simulink model "sampleModel7293_pp_1_1"  (R2018a)
settings: Solver=VariableStepAuto  StartTime=0.0  StopTime=10.0  RelTol=1e-3
undefined symbols (not defined in the file): DiscIntNeverNeededParam
libraries: simulink x367
(part 8 of 12)

== system sampleModel7293_pp_1_1/cfblk185/cfblk19 ==
  cfblk1 : Inport
  Action Port : ActionPort  ActionType=else
  cfblk3 : Delay  DelayLengthSource=Input port
      settings: InputPortMap=u0,p1
  cfblk4 : Subsystem  TreatAsAtomicUnit=on
  cfblk5 : DiscreteFir
  cfblk6 : simulink/Discrete/Transfer Fcn Lead or Lag  PoleZ=0.95  ZeroZ=0.75  ICPrevOutput=0.0  ICPrevInput=0.0  DoSatur=off
      settings: SourceProductName=Simulink  SourceProductBaseCode=SL
  cfblk7 : Subsystem  TreatAsAtomicUnit=on
  cfblk8 : Delay
  cyemi_{608..615} (8 alike) : DataTypeConversion  OutDataTypeStr=double
  emi_1381 : Subsystem  TreatAsAtomicUnit=on
  emi_1383 : If  IfExpression=0 <= u1
  emi_1384 : DataTypeConversion  OutDataTypeStr=double
  emi_1759 : Subsystem  TreatAsAtomicUnit=on
  emi_1761 : If  IfExpression=0 <= u1
  emi_1762 : DataTypeConversion  OutDataTypeStr=double
  cfblk2 : Outport
  wires:
  cfblk6/1 -> cfblk2/1, cyemi_611/1
  cfblk1/1 -> cyemi_613/1, cyemi_614/1
  cyemi_608/1 -> cfblk3/1
  cfblk8/1 -> cyemi_608/1, emi_1384/1
  cyemi_609/1 -> cfblk3/2
  cfblk3/1 -> cyemi_610/1
  cyemi_612/1 -> cfblk5/1
  cyemi_613/1 -> cfblk6/1
  cyemi_615/1 -> cfblk8/1
  cfblk5/1 -> cyemi_615/1, emi_1762/1
  cyemi_614/1 -> cfblk7/1(emi_1379)
  cfblk7/1(emi_1380) -> cyemi_609/1
  emi_1383/1 -> cfblk7/Action
  emi_1383/2 -> emi_1381/Action
  emi_1384/1 -> emi_1383/1
  cyemi_610/1 -> cfblk4/1(emi_1756)
  cyemi_611/1 -> cfblk4/2(emi_1757)
  cfblk4/1(emi_1758) -> cyemi_612/1
  emi_1761/1 -> cfblk4/Action
  emi_1761/2 -> emi_1759/Action
  emi_1762/1 -> emi_1761/1

== system sampleModel7293_pp_1_1/cfblk187/cfblk11 ==
  cfblk1 : Inport
  cfblk13 : Inport  Port=2
  cfblk14 : Inport  Port=3
  Action Port : ActionPort  ActionType=then
  cfblk10 : DiscreteFir
  cfblk11 : Delay  ShowEnablePort=on
      settings: InputPortMap=u0,e6
  cfblk12 : Subsystem  TreatAsAtomicUnit=on
  cfblk15 : Subsystem  TreatAsAtomicUnit=on
  cfblk3 : Subsystem  TreatAsAtomicUnit=on
  cfblk4 : Delay
  cfblk5 : DiscreteIntegrator  SampleTime=-1  OutDataTypeStr=double  ICPrevOutput=DiscIntNeverNeededParam  ICPrevScaledInput=DiscIntNeverNeededParam
  cfblk6 : UnitDelay  SampleTime=-1
  cfblk7 : DiscreteTransferFcn
  cfblk8 : simulink/Discrete/Transfer Fcn Lead or Lag  PoleZ=0.95  ZeroZ=0.75  ICPrevOutput=0.0  ICPrevInput=0.0  DoSatur=off
      settings: SourceProductName=Simulink  SourceProductBaseCode=SL
  cfblk9 : Subsystem  TreatAsAtomicUnit=on
  cyemi_{639..650} (12 alike) : DataTypeConversion  OutDataTypeStr=double
  emi_1353 : Subsystem  TreatAsAtomicUnit=on
  emi_{722,1355,1540,2009} (4 alike) : If  IfExpression=Inf <= u1
  emi_{723,1356,1541,2010} (4 alike) : DataTypeConversion  OutDataTypeStr=double
  emi_1538 : Subsystem  TreatAsAtomicUnit=on
  emi_2007 : Subsystem  TreatAsAtomicUnit=on
  emi_720 : Subsystem  TreatAsAtomicUnit=on
  cfblk2 : Outport
  wires:
  cfblk8/1 -> cfblk2/1
  cyemi_639/1 -> cfblk10/1
  cfblk11/1 -> cyemi_639/1, emi_1356/1
  cyemi_640/1 -> cfblk11/1
  cfblk6/1 -> cyemi_640/1
  cyemi_641/1 -> cfblk11/2
  cfblk5/1 -> cyemi_641/1, emi_1541/1
  cfblk7/1 -> cyemi_643/1
  cyemi_645/1 -> cfblk4/1
  cfblk13/1 -> cyemi_645/1
  cyemi_646/1 -> cfblk5/1
  cyemi_647/1 -> cfblk6/1
  cfblk1/1 -> cyemi_647/1
  cyemi_648/1 -> cfblk7/1
  cyemi_649/1 -> cfblk8/1
  cfblk14/1 -> cyemi_649/1
  cfblk4/1 -> cyemi_650/1
  cyemi_643/1 -> cfblk15/1(emi_718)
  cfblk15/1(emi_719) -> cyemi_644/1, emi_2010/1
  emi_722/1 -> cfblk15/Action
  emi_722/2 -> emi_720/Action
  emi_723/1 -> emi_722/1
  cyemi_642/1 -> cfblk12/1(emi_1351)
  cfblk12/1(emi_1352) -> cyemi_646/1
  emi_1355/1 -> cfblk12/Action
  emi_1355/2 -> emi_1353/Action
  emi_1356/1 -> emi_1355/1
  cyemi_650/1 -> cfblk9/1(emi_1536)
  cfblk9/1(emi_1537) -> cyemi_642/1
  emi_1540/1 -> cfblk9/Action
  emi_1540/2 -> emi_1538/Action
  emi_1541/1 -> emi_1540/1
  cyemi_644/1 -> cfblk3/1(emi_2005)
  cfblk3/1(emi_2006) -> emi_723/1, cyemi_648/1
  emi_2009/1 -> cfblk3/Action
  emi_2009/2 -> emi_2007/Action
  emi_2010/1 -> emi_2009/1

== system sampleModel7293_pp_1_1/cfblk187/cfblk12 ==
  cfblk1 : Inport
  cfblk8 : Inport  Port=2
  cfblk9 : Inport  Port=3
  Action Port : ActionPort  ActionType=else
  cfblk3 : Subsystem  TreatAsAtomicUnit=on
  cfblk4 : DiscreteIntegrator  SampleTime=-1  OutDataTypeStr=double  ICPrevOutput=DiscIntNeverNeededParam  ICPrevScaledInput=DiscIntNeverNeededParam
  cfblk5 : Delay
  cfblk6 : DiscreteZeroPole  Poles=[0 0.5]  Gain=1  SampleTime=-1
  cfblk7 : Subsystem  TreatAsAtomicUnit=on
  cyemi_{654..659} (6 alike) : DataTypeConversion  OutDataTypeStr=double
  emi_1190 : Subsystem  TreatAsAtomicUnit=on
  emi_1192 : If  IfExpression=0 <= u1
  emi_1193 : DataTypeConversion  OutDataTypeStr=double
  emi_324 : Subsystem  TreatAsAtomicUnit=on
  emi_326 : If  IfExpression=0 <= u1
  emi_327 : DataTypeConversion  OutDataTypeStr=double
  cfblk2 : Outport
  cfblk10 : Outport  Port=2
  wires:
  cfblk5/1 -> cfblk2/1
  cfblk8/1 -> cfblk10/1
  cfblk1/1 -> cyemi_654/1
  cfblk6/1 -> cyemi_655/1, emi_327/1
  cyemi_656/1 -> cfblk4/1
  cyemi_657/1 -> cfblk5/1
  cyemi_658/1 -> cfblk6/1
  cfblk4/1 -> cyemi_658/1, emi_1193/1
  cfblk9/1 -> cyemi_659/1
  cyemi_659/1 -> cfblk7/1(emi_322)
  cfblk7/1(emi_323) -> cyemi_656/1
  emi_326/1 -> cfblk7/Action
  emi_326/2 -> emi_324/Action
  emi_327/1 -> emi_326/1
  cyemi_654/1 -> cfblk3/1(emi_1187)
  cyemi_655/1 -> cfblk3/2(emi_1188)
  cfblk3/1(emi_1189) -> cyemi_657/1
  emi_1192/1 -> cfblk3/Action
  emi_1192/2 -> emi_1190/Action
  emi_1193/1 -> emi_1192/1

== system sampleModel7293_pp_1_1/cfblk187/cfblk14 ==
  emi_774 : Inport
  Action Port : ActionPort  ActionType=then
  cfblk14 : Delay
  emi_775 : Outport
  wires:
  emi_774/1 -> cfblk14/1
  cfblk14/1 -> emi_775/1

== system sampleModel7293_pp_1_1/cfblk187/cfblk3 ==
  emi_336 : Inport
  emi_337 : Inport  Port=2
  Action Port : ActionPort  ActionType=then
  cfblk3 : simulink/Continuous/PID Controller (2DOF)  Controller=PID  TimeDomain=Discrete-time  SampleTime=-1  IntegratorMethod=Forward Euler  FilterMethod=Forward Euler  Form=Parallel  UseFilter=on  ControllerParametersSource=internal  P=1  I=1  D=0  N=100  b=1  c=1  InitialConditionSource=internal  InitialConditionForIntegrator=0  InitialConditionForFilter=0  ExternalReset=none  LimitOutput=off  UpperSaturationLimit=inf  LowerSaturationLimit=-inf  LinearizeAsGain=off  AntiWindupMode=none  Kb=1  TrackingMode=off  Kt=1  PParamMin=[]  PParamMax=[]  IParamMin=[]  IParamMax=[]  DParamMin=[]  DParamMax=[]  NParamMin=[]  NParamMax=[]  bParamMin=[]  bParamMax=[]  cParamMin=[]  cParamMax=[]  KbParamMin=[]  KbParamMax=[]  KtParamMin=[]  KtParamMax=[]  POutMin=[]  POutMax=[]  IOutMin=[]  IOutMax=[]  DOutMin=[]  DOutMax=[]  NOutMin=[]  NOutMax=[]  bOutMin=[]  bOutMax=[]  cOutMin=[]  cOutMax=[]  KbOutMin=[]  KbOutMax=[]  KtOutMin=[]  KtOutMax=[]  IntegratorOutMin=[]  IntegratorOutMax=[]  FilterOutMin=[]  FilterOutMax=[]  SumOutMin=[]  SumOutMax=[]  Sum1OutMin=[]  Sum1OutMax=[]  Sum2OutMin=[]  Sum2OutMax=[]  Sum3OutMin=[]  Sum3OutMax=[]  SumI1OutMin=[]  SumI1OutMax=[]  SumI2OutMin=[]  SumI2OutMax=[]  SumI3OutMin=[]  SumI3OutMax=[]  SumDOutMin=[]  SumDOutMax=[]  SaturationOutMin=[]  SaturationOutMax=[]  IntegratorContinuousStateAttributes=''  IntegratorStateMustResolveToSignalObject=off  IntegratorRTWStateStorageClass=Auto  FilterContinuousStateAttributes=''  FilterStateMustResolveToSignalObject=off  FilterRTWStateStorageClass=Auto  DifferentiatorICPrevScaledInput=0  DifferentiatorOutMin=[]  DifferentiatorOutMax=[]  FilterDiffOutCoefMin=[]  FilterDiffOutCoefMax=[]  SumDenOutMin=[]  SumDenOutMax=[]  SumNumOutMin=[]  SumNumOutMax=[]  ReciprocalOutMin=[]  ReciprocalOutMax=[]  DivideOutMin=[]  DivideOutMax=[]  TunerSelectOption=Transfer Function Based (PID Tuner App)
  emi_338 : Outport
  wires:
  emi_336/1 -> cfblk3/1
  emi_337/1 -> cfblk3/2
  cfblk3/1 -> emi_338/1

== system sampleModel7293_pp_1_1/cfblk187/emi_339 ==
  Action Port : ActionPort  ActionType=else
  emi_340 : Assertion

== system sampleModel7293_pp_1_1/cfblk187/emi_776 ==
  Action Port : ActionPort  ActionType=else
  emi_777 : Assertion

== system sampleModel7293_pp_1_1/cfblk188/cfblk3 ==
  emi_646 : Inport
  Action Port : ActionPort  ActionType=then
  cfblk3 : DiscreteTransferFcn
  emi_647 : Outport
  wires:
  emi_646/1 -> cfblk3/1
  cfblk3/1 -> emi_647/1

== system sampleModel7293_pp_1_1/cfblk188/cfblk4 ==
  emi_1471 : Inport
  Action Port : ActionPort  ActionType=then
  cfblk4 : DiscreteFir
  emi_1472 : Outport
  wires:
  emi_1471/1 -> cfblk4/1
  cfblk4/1 -> emi_1472/1

== system sampleModel7293_pp_1_1/cfblk188/cfblk5 ==
  emi_450 : Inport
  Action Port : ActionPort  ActionType=then
  cfblk5 : DiscreteZeroPole  Poles=[0 0.5]  Gain=1  SampleTime=-1
  emi_451 : Outport
  wires:
  emi_450/1 -> cfblk5/1
  cfblk5/1 -> emi_451/1

== system sampleModel7293_pp_1_1/cfblk188/cfblk6 ==
  emi_178 : Inport
  Action Port : ActionPort  ActionType=then
  cfblk6 : simulink/Discrete/Transfer Fcn First Order  PoleZ=0.95  ICPrevOutput=0.0  DoSatur=off
      settings: SourceProductName=Simulink
  emi_179 : Outport
  wires:
  emi_178/1 -> cfblk6/1
  cfblk6/1 -> emi_179/1

== system sampleModel7293_pp_1_1/cfblk188/emi_1473 ==
  Action Port : ActionPort  ActionType=else
  emi_1474 : Assertion

== system sampleModel7293_pp_1_1/cfblk188/emi_180 ==
  Action Port : ActionPort  ActionType=else
  emi_181 : Assertion

== system sampleModel7293_pp_1_1/cfblk188/emi_452 ==
  Action Port : ActionPort  ActionType=else
  emi_453 : Assertion

== system sampleModel7293_pp_1_1/cfblk188/emi_648 ==
  Action Port : ActionPort  ActionType=else
  emi_649 : Assertion

== system sampleModel7293_pp_1_1/cfblk189/cfblk16 ==
  cfblk1 : Inport
  cfblk11 : Inport  Port=2
  cfblk12 : Inport  Port=3
  cfblk13 : Inport  Port=4
  Action Port : ActionPort  ActionType=then
  cfblk10 : simulink/Continuous/PID Controller (2DOF)  Controller=PID  TimeDomain=Discrete-time  SampleTime=-1  IntegratorMethod=Forward Euler  FilterMethod=Forward Euler  Form=Parallel  UseFilter=on  ControllerParametersSource=internal  P=1  I=1  D=0  N=100  b=1  c=1  InitialConditionSource=internal  InitialConditionForIntegrator=0  InitialConditionForFilter=0  ExternalReset=none  LimitOutput=off  UpperSaturationLimit=inf  LowerSaturationLimit=-inf  LinearizeAsGain=off  AntiWindupMode=none  Kb=1  TrackingMode=off  Kt=1  PParamMin=[]  PParamMax=[]  IParamMin=[]  IParamMax=[]  DParamMin=[]  DParamMax=[]  NParamMin=[]  NParamMax=[]  bParamMin=[]  bParamMax=[]  cParamMin=[]  cParamMax=[]  KbParamMin=[]  KbParamMax=[]  KtParamMin=[]  KtParamMax=[]  POutMin=[]  POutMax=[]  IOutMin=[]  IOutMax=[]  DOutMin=[]  DOutMax=[]  NOutMin=[]  NOutMax=[]  bOutMin=[]  bOutMax=[]  cOutMin=[]  cOutMax=[]  KbOutMin=[]  KbOutMax=[]  KtOutMin=[]  KtOutMax=[]  IntegratorOutMin=[]  IntegratorOutMax=[]  FilterOutMin=[]  FilterOutMax=[]  SumOutMin=[]  SumOutMax=[]  Sum1OutMin=[]  Sum1OutMax=[]  Sum2OutMin=[]  Sum2OutMax=[]  Sum3OutMin=[]  Sum3OutMax=[]  SumI1OutMin=[]  SumI1OutMax=[]  SumI2OutMin=[]  SumI2OutMax=[]  SumI3OutMin=[]  SumI3OutMax=[]  SumDOutMin=[]  SumDOutMax=[]  SaturationOutMin=[]  SaturationOutMax=[]  IntegratorContinuousStateAttributes=''  IntegratorStateMustResolveToSignalObject=off  IntegratorRTWStateStorageClass=Auto  FilterContinuousStateAttributes=''  FilterStateMustResolveToSignalObject=off  FilterRTWStateStorageClass=Auto  DifferentiatorICPrevScaledInput=0  DifferentiatorOutMin=[]  DifferentiatorOutMax=[]  FilterDiffOutCoefMin=[]  FilterDiffOutCoefMax=[]  SumDenOutMin=[]  SumDenOutMax=[]  SumNumOutMin=[]  SumNumOutMax=[]  ReciprocalOutMin=[]  ReciprocalOutMax=[]  DivideOutMin=[]  DivideOutMax=[]  TunerSelectOption=Transfer Function Based (PID Tuner App)
  cfblk3 : DiscreteFilter
  cfblk4 : simulink/Discrete/Transfer Fcn Real Zero  ZeroZ=0.75  ICPrevInput=0.0  DoSatur=off
      settings: SourceProductName=Simulink  SourceProductBaseCode=SL
  cfblk5 : simulink/Discrete/Tapped Delay  vinit=0.0  samptime=-1  NumDelays=1  DelayOrder=Oldest  includeCurrent=off
  cfblk6 : simulink/Discrete/Difference  ICPrevInput=0.0  OutMin=[]  OutMax=[]  OutDataTypeStr=double  OutputDataTypeScalingMode=double  OutDataType=fixdt(1, 16)  OutScaling=2^-10  DoSatur=off
  cfblk7 : simulink/Discrete/Transfer Fcn Lead or Lag  PoleZ=0.95  ZeroZ=0.75  ICPrevOutput=0.0  ICPrevInput=0.0  DoSatur=off
      settings: SourceProductName=Simulink  SourceProductBaseCode=SL
  cfblk8 : Subsystem  TreatAsAtomicUnit=on
  cfblk9 : DiscreteZeroPole  Poles=[0 0.5]  Gain=1  SampleTime=-1
  cyemi_{690..698} (9 alike) : DataTypeConversion  OutDataTypeStr=double
  emi_905 : Subsystem  TreatAsAtomicUnit=on
  emi_907 : If  IfExpression=0 <= u1
  emi_908 : DataTypeConversion  OutDataTypeStr=double
  cfblk2 : Outport
  wires:
  cfblk9/1 -> cfblk2/1
  cyemi_690/1 -> cfblk10/1
  cfblk6/1 -> cyemi_690/1
  cyemi_691/1 -> cfblk10/2
  cfblk7/1 -> cyemi_691/1
  cyemi_692/1 -> cfblk3/1
  cfblk12/1 -> cyemi_692/1
  cyemi_693/1 -> cfblk4/1
  cfblk11/1 -> cyemi_693/1
  cyemi_694/1 -> cfblk5/1
  cfblk4/1 -> cyemi_694/1
  cyemi_695/1 -> cfblk6/1
  cyemi_696/1 -> cfblk7/1
  cfblk13/1 -> cyemi_696/1
  cfblk3/1 -> cyemi_697/1, emi_908/1
  cyemi_698/1 -> cfblk9/1
  cfblk1/1 -> cyemi_698/1
  cyemi_697/1 -> cfblk8/1(emi_903)
  cfblk8/1(emi_904) -> cyemi_695/1
  emi_907/1 -> cfblk8/Action
  emi_907/2 -> emi_905/Action
  emi_908/1 -> emi_907/1

== system sampleModel7293_pp_1_1/cfblk189/cfblk17 ==
  cfblk1 : Inport
  cfblk15 : Inport  Port=2
  Action Port : ActionPort  ActionType=else
  cfblk10 : simulink/Continuous/PID Controller  Controller=PID  TimeDomain=Discrete-time  SampleTime=-1  IntegratorMethod=Forward Euler  FilterMethod=Forward Euler  Form=Parallel  UseFilter=on  ControllerParametersSource=internal  P=1  I=1  D=0  N=100  InitialConditionSource=internal  InitialConditionForIntegrator=0  InitialConditionForFilter=0  ExternalReset=none  LimitOutput=off  UpperSaturationLimit=inf  LowerSaturationLimit=-inf  LinearizeAsGain=off  AntiWindupMode=none  Kb=1  TrackingMode=off  Kt=1  PParamMin=[]  PParamMax=[]  IParamMin=[]  IParamMax=[]  DParamMin=[]  DParamMax=[]  NParamMin=[]  NParamMax=[]  KbParamMin=[]  KbParamMax=[]  KtParamMin=[]  KtParamMax=[]  POutMin=[]  POutMax=[]  IOutMin=[]  IOutMax=[]  DOutMin=[]  DOutMax=[]  NOutMin=[]  NOutMax=[]  KbOutMin=[]  KbOutMax=[]  KtOutMin=[]  KtOutMax=[]  IntegratorOutMin=[]  IntegratorOutMax=[]  FilterOutMin=[]  FilterOutMax=[]  SumOutMin=[]  SumOutMax=[]  SumI1OutMin=[]  SumI1OutMax=[]  SumI2OutMin=[]  SumI2OutMax=[]  SumI3OutMin=[]  SumI3OutMax=[]  SumDOutMin=[]  SumDOutMax=[]  SaturationOutMin=[]  SaturationOutMax=[]  IntegratorContinuousStateAttributes=''  IntegratorStateMustResolveToSignalObject=off  IntegratorRTWStateStorageClass=Auto  FilterContinuousStateAttributes=''  FilterStateMustResolveToSignalObject=off  FilterRTWStateStorageClass=Auto  DifferentiatorICPrevScaledInput=0  DifferentiatorOutMin=[]  DifferentiatorOutMax=[]  FilterDiffOutCoefMin=[]  FilterDiffOutCoefMax=[]  SumDenOutMin=[]  SumDenOutMax=[]  SumNumOutMin=[]  SumNumOutMax=[]  ReciprocalOutMin=[]  ReciprocalOutMax=[]  DivideOutMin=[]  DivideOutMax=[]  TunerSelectOption=Transfer Function Based (PID Tuner App)
  cfblk11 : simulink/Discrete/Tapped Delay  vinit=0.0  samptime=-1  NumDelays=1  DelayOrder=Oldest  includeCurrent=off
  cfblk12 : DiscreteFilter
  cfblk13 : Subsystem  TreatAsAtomicUnit=on
  cfblk14 : DiscreteStateSpace  SampleTime=-1
  cfblk16 : Delay
  cfblk17 : DataTypeConversion  OutDataTypeStr=uint32
  cfblk3 : DiscreteTransferFcn
  cfblk4 : Subsystem  TreatAsAtomicUnit=on
  cfblk5 : Delay  ShowEnablePort=on
      settings: InputPortMap=u0,e6
  cfblk6 : simulink/Discrete/Transfer Fcn Lead or Lag  PoleZ=0.95  ZeroZ=0.75  ICPrevOutput=0.0  ICPrevInput=0.0  DoSatur=off
      settings: SourceProductName=Simulink  SourceProductBaseCode=SL
  cfblk7 : simulink/Continuous/PID Controller  Controller=PID  TimeDomain=Discrete-time  SampleTime=-1  IntegratorMethod=Forward Euler  FilterMethod=Forward Euler  Form=Parallel  UseFilter=on  ControllerParametersSource=internal  P=1  I=1  D=0  N=100  InitialConditionSource=internal  InitialConditionForIntegrator=0  InitialConditionForFilter=0  ExternalReset=none  LimitOutput=off  UpperSaturationLimit=inf  LowerSaturationLimit=-inf  LinearizeAsGain=off  AntiWindupMode=none  Kb=1  TrackingMode=off  Kt=1  PParamMin=[]  PParamMax=[]  IParamMin=[]  IParamMax=[]  DParamMin=[]  DParamMax=[]  NParamMin=[]  NParamMax=[]  KbParamMin=[]  KbParamMax=[]  KtParamMin=[]  KtParamMax=[]  POutMin=[]  POutMax=[]  IOutMin=[]  IOutMax=[]  DOutMin=[]  DOutMax=[]  NOutMin=[]  NOutMax=[]  KbOutMin=[]  KbOutMax=[]  KtOutMin=[]  KtOutMax=[]  IntegratorOutMin=[]  IntegratorOutMax=[]  FilterOutMin=[]  FilterOutMax=[]  SumOutMin=[]  SumOutMax=[]  SumI1OutMin=[]  SumI1OutMax=[]  SumI2OutMin=[]  SumI2OutMax=[]  SumI3OutMin=[]  SumI3OutMax=[]  SumDOutMin=[]  SumDOutMax=[]  SaturationOutMin=[]  SaturationOutMax=[]  IntegratorContinuousStateAttributes=''  IntegratorStateMustResolveToSignalObject=off  IntegratorRTWStateStorageClass=Auto  FilterContinuousStateAttributes=''  FilterStateMustResolveToSignalObject=off  FilterRTWStateStorageClass=Auto  DifferentiatorICPrevScaledInput=0  DifferentiatorOutMin=[]  DifferentiatorOutMax=[]  FilterDiffOutCoefMin=[]  FilterDiffOutCoefMax=[]  SumDenOutMin=[]  SumDenOutMax=[]  SumNumOutMin=[]  SumNumOutMax=[]  ReciprocalOutMin=[]  ReciprocalOutMax=[]  DivideOutMin=[]  DivideOutMax=[]  TunerSelectOption=Transfer Function Based (PID Tuner App)
  cfblk8 : simulink/Continuous/PID Controller  Controller=PID  TimeDomain=Discrete-time  SampleTime=-1  IntegratorMethod=Forward Euler  FilterMethod=Forward Euler  Form=Parallel  UseFilter=on  ControllerParametersSource=internal  P=1  I=1  D=0  N=100  InitialConditionSource=internal  InitialConditionForIntegrator=0  InitialConditionForFilter=0  ExternalReset=none  LimitOutput=off  UpperSaturationLimit=inf  LowerSaturationLimit=-inf  LinearizeAsGain=off  AntiWindupMode=none  Kb=1  TrackingMode=off  Kt=1  PParamMin=[]  PParamMax=[]  IParamMin=[]  IParamMax=[]  DParamMin=[]  DParamMax=[]  NParamMin=[]  NParamMax=[]  KbParamMin=[]  KbParamMax=[]  KtParamMin=[]  KtParamMax=[]  POutMin=[]  POutMax=[]  IOutMin=[]  IOutMax=[]  DOutMin=[]  DOutMax=[]  NOutMin=[]  NOutMax=[]  KbOutMin=[]  KbOutMax=[]  KtOutMin=[]  KtOutMax=[]  IntegratorOutMin=[]  IntegratorOutMax=[]  FilterOutMin=[]  FilterOutMax=[]  SumOutMin=[]  SumOutMax=[]  SumI1OutMin=[]  SumI1OutMax=[]  SumI2OutMin=[]  SumI2OutMax=[]  SumI3OutMin=[]  SumI3OutMax=[]  SumDOutMin=[]  SumDOutMax=[]  SaturationOutMin=[]  SaturationOutMax=[]  IntegratorContinuousStateAttributes=''  IntegratorStateMustResolveToSignalObject=off  IntegratorRTWStateStorageClass=Auto  FilterContinuousStateAttributes=''  FilterStateMustResolveToSignalObject=off  FilterRTWStateStorageClass=Auto  DifferentiatorICPrevScaledInput=0  DifferentiatorOutMin=[]  DifferentiatorOutMax=[]  FilterDiffOutCoefMin=[]  FilterDiffOutCoefMax=[]  SumDenOutMin=[]  SumDenOutMax=[]  SumNumOutMin=[]  SumNumOutMax=[]  ReciprocalOutMin=[]  ReciprocalOutMax=[]  DivideOutMin=[]  DivideOutMax=[]  TunerSelectOption=Transfer Function Based (PID Tuner App)
  cfblk9 : Subsystem  TreatAsAtomicUnit=on
  cyemi_{701..715} (15 alike) : DataTypeConversion  OutDataTypeStr=double
  emi_361 : Subsystem  TreatAsAtomicUnit=on
  emi_363 : If  IfExpression=0 <= u1
  emi_364 : DataTypeConversion  OutDataTypeStr=double
  emi_368 : Subsystem  TreatAsAtomicUnit=on
  emi_370 : If  IfExpression=0 <= u1
  emi_371 : DataTypeConversion  OutDataTypeStr=double
  emi_812 : Subsystem  TreatAsAtomicUnit=on
  emi_814 : If  IfExpression=0 <= u1
  emi_815 : DataTypeConversion  OutDataTypeStr=double
  cfblk2 : Outport
  wires:
  cfblk17/1 -> cfblk2/1
  cyemi_701/1 -> cfblk10/1
  cfblk11/1 -> cyemi_701/1, emi_815/1
  cyemi_702/1 -> cfblk11/1
  cfblk12/1 -> cyemi_702/1
  cyemi_703/1 -> cfblk12/1
  cfblk7/1 -> cyemi_703/1
  cfblk10/1 -> cyemi_704/1
  cyemi_705/1 -> cfblk14/1
  cfblk15/1 -> cyemi_705/1
  cyemi_706/1 -> cfblk16/1
  cyemi_707/1 -> cfblk17/1
  cyemi_708/1 -> cfblk3/1
  cfblk8/1 -> cyemi_708/1
  cfblk14/1 -> cyemi_709/1
  cyemi_710/1 -> cfblk5/1
  cyemi_711/1 -> cfblk5/2
  cfblk16/1 -> cyemi_711/1
  cyemi_712/1 -> cfblk6/1
  cfblk5/1 -> cyemi_712/1
  cyemi_713/1 -> cfblk7/1
  cfblk6/1 -> cyemi_713/1
  cyemi_714/1 -> cfblk8/1
  cfblk1/1 -> cyemi_714/1
  cfblk3/1 -> cyemi_715/1, emi_364/1, emi_371/1
  cyemi_704/1 -> cfblk13/1(emi_359)
  cfblk13/1(emi_360) -> cyemi_706/1
  emi_363/1 -> cfblk13/Action
  emi_363/2 -> emi_361/Action
  emi_364/1 -> emi_363/1
  cyemi_715/1 -> cfblk9/1(emi_366)
  cfblk9/1(emi_367) -> cyemi_710/1
  emi_370/1 -> cfblk9/Action
  emi_370/2 -> emi_368/Action
  emi_371/1 -> emi_370/1
  cyemi_709/1 -> cfblk4/1(emi_810)
  cfblk4/1(emi_811) -> cyemi_707/1
  emi_814/1 -> cfblk4/Action
  emi_814/2 -> emi_812/Action
  emi_815/1 -> emi_814/1

== system sampleModel7293_pp_1_1/cfblk189/cfblk4 ==
  emi_1237 : Inport
  emi_1238 : Inport  Port=2
  Action Port : ActionPort  ActionType=then
  cfblk4 : simulink/Continuous/PID Controller (2DOF)  Controller=PID  TimeDomain=Discrete-time  SampleTime=-1  IntegratorMethod=Forward Euler  FilterMethod=Forward Euler  Form=Parallel  UseFilter=on  ControllerParametersSource=internal  P=1  I=1  D=0  N=100  b=1  c=1  InitialConditionSource=internal  InitialConditionForIntegrator=0  InitialConditionForFilter=0  ExternalReset=none  LimitOutput=off  UpperSaturationLimit=inf  LowerSaturationLimit=-inf  LinearizeAsGain=off  AntiWindupMode=none  Kb=1  TrackingMode=off  Kt=1  PParamMin=[]  PParamMax=[]  IParamMin=[]  IParamMax=[]  DParamMin=[]  DParamMax=[]  NParamMin=[]  NParamMax=[]  bParamMin=[]  bParamMax=[]  cParamMin=[]  cParamMax=[]  KbParamMin=[]  KbParamMax=[]  KtParamMin=[]  KtParamMax=[]  POutMin=[]  POutMax=[]  IOutMin=[]  IOutMax=[]  DOutMin=[]  DOutMax=[]  NOutMin=[]  NOutMax=[]  bOutMin=[]  bOutMax=[]  cOutMin=[]  cOutMax=[]  KbOutMin=[]  KbOutMax=[]  KtOutMin=[]  KtOutMax=[]  IntegratorOutMin=[]  IntegratorOutMax=[]  FilterOutMin=[]  FilterOutMax=[]  SumOutMin=[]  SumOutMax=[]  Sum1OutMin=[]  Sum1OutMax=[]  Sum2OutMin=[]  Sum2OutMax=[]  Sum3OutMin=[]  Sum3OutMax=[]  SumI1OutMin=[]  SumI1OutMax=[]  SumI2OutMin=[]  SumI2OutMax=[]  SumI3OutMin=[]  SumI3OutMax=[]  SumDOutMin=[]  SumDOutMax=[]  SaturationOutMin=[]  SaturationOutMax=[]  IntegratorContinuousStateAttributes=''  IntegratorStateMustResolveToSignalObject=off  IntegratorRTWStateStorageClass=Auto  FilterContinuousStateAttributes=''  FilterStateMustResolveToSignalObject=off  FilterRTWStateStorageClass=Auto  DifferentiatorICPrevScaledInput=0  DifferentiatorOutMin=[]  DifferentiatorOutMax=[]  FilterDiffOutCoefMin=[]  FilterDiffOutCoefMax=[]  SumDenOutMin=[]  SumDenOutMax=[]  SumNumOutMin=[]  SumNumOutMax=[]  ReciprocalOutMin=[]  ReciprocalOutMax=[]  DivideOutMin=[]  DivideOutMax=[]  TunerSelectOption=Transfer Function Based (PID Tuner App)
  emi_1239 : Outport
  wires:
  emi_1237/1 -> cfblk4/1
  emi_1238/1 -> cfblk4/2
  cfblk4/1 -> emi_1239/1

== system sampleModel7293_pp_1_1/cfblk189/cfblk5 ==
  emi_1508 : Inport
  Action Port : ActionPort  ActionType=then
  cfblk5 : simulink/Discrete/Transfer Fcn Lead or Lag  PoleZ=0.95  ZeroZ=0.75  ICPrevOutput=0.0  ICPrevInput=0.0  DoSatur=off
      settings: SourceProductName=Simulink  SourceProductBaseCode=SL
  emi_1509 : Outport
  wires:
  emi_1508/1 -> cfblk5/1
  cfblk5/1 -> emi_1509/1

== system sampleModel7293_pp_1_1/cfblk189/emi_1240 ==
  Action Port : ActionPort  ActionType=else
  emi_1241 : Assertion

== system sampleModel7293_pp_1_1/cfblk189/emi_1510 ==
  Action Port : ActionPort  ActionType=else
  emi_1511 : Assertion

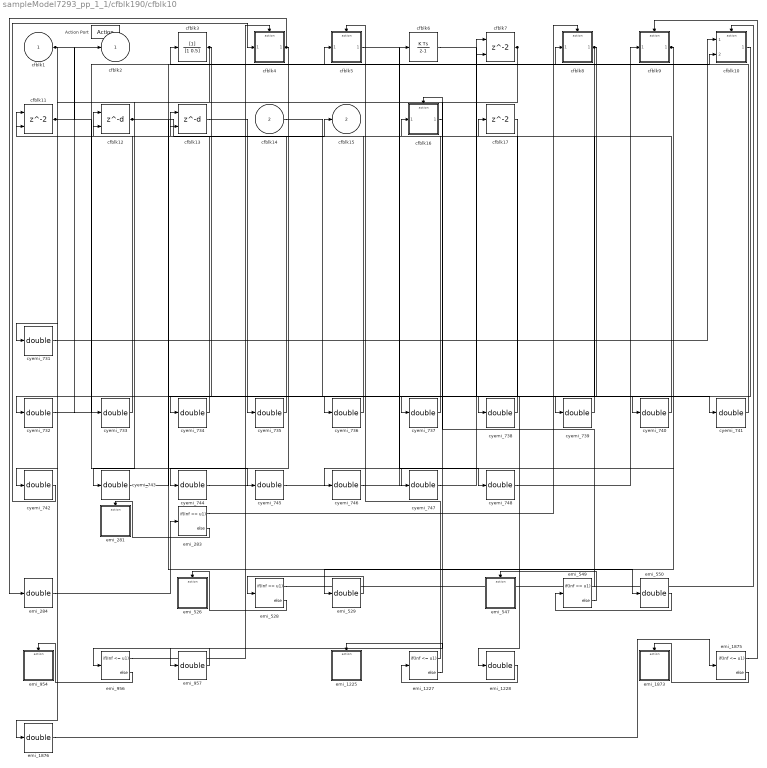
== system sampleModel7293_pp_1_1/cfblk190/cfblk10 ==
  cfblk1 : Inport
  cfblk14 : Inport  Port=2
  Action Port : ActionPort  ActionType=else
  cfblk10 : Subsystem  TreatAsAtomicUnit=on
  cfblk11 : Delay  ShowEnablePort=on
      settings: InputPortMap=u0,e6
  cfblk12 : Delay  DelayLengthSource=Input port
      settings: InputPortMap=u0,p1
  cfblk13 : Delay  DelayLengthSource=Input port
      settings: InputPortMap=u0,p1
  cfblk16 : Subsystem  TreatAsAtomicUnit=on
  cfblk17 : Delay
  cfblk3 : DiscreteFilter
  cfblk4 : Subsystem  TreatAsAtomicUnit=on
  cfblk5 : Subsystem  TreatAsAtomicUnit=on
  cfblk6 : DiscreteIntegrator  SampleTime=-1  OutDataTypeStr=double  ICPrevOutput=DiscIntNeverNeededParam  ICPrevScaledInput=DiscIntNeverNeededParam
  cfblk7 : Delay  ShowEnablePort=on
      settings: InputPortMap=u0,e6
  cfblk8 : Subsystem  TreatAsAtomicUnit=on
  cfblk9 : Subsystem  TreatAsAtomicUnit=on
  cyemi_{731..748} (18 alike) : DataTypeConversion  OutDataTypeStr=double
  emi_1225 : Subsystem  TreatAsAtomicUnit=on
  emi_{283,528,549,956,1227,1875} (6 alike) : If  IfExpression=Inf <= u1
  emi_{284,529,550,957,1228,1876} (6 alike) : DataTypeConversion  OutDataTypeStr=double
  emi_1873 : Subsystem  TreatAsAtomicUnit=on
  emi_281 : Subsystem  TreatAsAtomicUnit=on
  emi_526 : Subsystem  TreatAsAtomicUnit=on
  emi_547 : Subsystem  TreatAsAtomicUnit=on
  emi_954 : Subsystem  TreatAsAtomicUnit=on
  cfblk2 : Outport
  cfblk15 : Outport  Port=2
  wires:
  cfblk11/1 -> cfblk2/1, cyemi_745/1
  cfblk1/1 -> cyemi_731/1, cyemi_733/1
  cfblk3/1 -> cyemi_732/1, cyemi_734/1, emi_1876/1
  cfblk12/1 -> cfblk15/1, cyemi_739/1, emi_550/1
  cyemi_733/1 -> cfblk11/1
  cyemi_734/1 -> cfblk11/2
  cyemi_735/1 -> cfblk12/1
  cfblk13/1 -> cyemi_735/1
  cyemi_736/1 -> cfblk12/2
  cyemi_737/1 -> cfblk13/1
  cyemi_738/1 -> cfblk13/2
  cyemi_740/1 -> cfblk17/1
  cfblk6/1 -> cyemi_740/1
  cyemi_741/1 -> cfblk3/1
  cfblk14/1 -> cyemi_741/1
  cfblk17/1 -> cyemi_742/1
  cfblk7/1 -> cyemi_743/1, emi_957/1
  cyemi_744/1 -> cfblk6/1
  cyemi_745/1 -> cfblk7/1
  cyemi_746/1 -> cfblk7/2
  cyemi_747/1 -> cfblk8/1(emi_279)
  cfblk8/1(emi_280) -> cyemi_737/1, cyemi_736/1, emi_1228/1
  emi_283/1 -> cfblk8/Action
  emi_283/2 -> emi_281/Action
  emi_284/1 -> emi_283/1
  cyemi_731/1 -> cfblk10/1(emi_523)
  cyemi_732/1 -> cfblk10/2(emi_524)
  cfblk10/1(emi_525) -> cyemi_738/1
  emi_528/1 -> cfblk10/Action
  emi_528/2 -> emi_526/Action
  emi_529/1 -> emi_528/1
  cyemi_739/1 -> cfblk16/1(emi_545)
  cfblk16/1(emi_546) -> cyemi_746/1
  emi_549/1 -> cfblk16/Action
  emi_549/2 -> emi_547/Action
  emi_550/1 -> emi_549/1
  cyemi_742/1 -> cfblk4/1(emi_952)
  cfblk4/1(emi_953) -> emi_284/1, cyemi_744/1
  emi_956/1 -> cfblk4/Action
  emi_956/2 -> emi_954/Action
  emi_957/1 -> emi_956/1
  cyemi_743/1 -> cfblk5/1(emi_1223)
  cfblk5/1(emi_1224) -> cyemi_748/1
  emi_1227/1 -> cfblk5/Action
  emi_1227/2 -> emi_1225/Action
  emi_1228/1 -> emi_1227/1
  cyemi_748/1 -> cfblk9/1(emi_1871)
  cfblk9/1(emi_1872) -> emi_529/1, cyemi_747/1
  emi_1875/1 -> cfblk9/Action
  emi_1875/2 -> emi_1873/Action
  emi_1876/1 -> emi_1875/1

== system sampleModel7293_pp_1_1/cfblk190/cfblk12 ==
  emi_2140 : Inport
  Action Port : ActionPort  ActionType=then
  cfblk12 : Delay
  emi_2141 : Outport
  wires:
  emi_2140/1 -> cfblk12/1
  cfblk12/1 -> emi_2141/1

== system sampleModel7293_pp_1_1/cfblk190/cfblk13 ==
  emi_1800 : Inport
  Action Port : ActionPort  ActionType=then
  cfblk13 : Delay
  emi_1801 : Outport
  wires:
  emi_1800/1 -> cfblk13/1
  cfblk13/1 -> emi_1801/1

== system sampleModel7293_pp_1_1/cfblk190/cfblk3 ==
  emi_2026 : Inport
  Action Port : ActionPort  ActionType=then
  cfblk3 : simulink/Discrete/Transfer Fcn Lead or Lag  PoleZ=0.95  ZeroZ=0.75  ICPrevOutput=0.0  ICPrevInput=0.0  DoSatur=off
      settings: SourceProductName=Simulink  SourceProductBaseCode=SL
  emi_2027 : Outport
  wires:
  emi_2026/1 -> cfblk3/1
  cfblk3/1 -> emi_2027/1

== system sampleModel7293_pp_1_1/cfblk190/cfblk5 ==
  emi_917 : Inport
  Action Port : ActionPort  ActionType=then
  cfblk5 : simulink/Discrete/Transfer Fcn Real Zero  ZeroZ=0.75  ICPrevInput=0.0  DoSatur=off
      settings: SourceProductName=Simulink  SourceProductBaseCode=SL
  emi_918 : Outport
  wires:
  emi_917/1 -> cfblk5/1
  cfblk5/1 -> emi_918/1

== system sampleModel7293_pp_1_1/cfblk190/cfblk9 ==
  cfblk1 : Inport
  Action Port : ActionPort  ActionType=then
  cfblk10 : Subsystem  TreatAsAtomicUnit=on
  cfblk11 : DiscreteZeroPole  Poles=[0 0.5]  Gain=1  SampleTime=-1
  cfblk12 : DiscreteTransferFcn
  cfblk13 : simulink/Continuous/PID Controller (2DOF)  Controller=PID  TimeDomain=Discrete-time  SampleTime=-1  IntegratorMethod=Forward Euler  FilterMethod=Forward Euler  Form=Parallel  UseFilter=on  ControllerParametersSource=internal  P=1  I=1  D=0  N=100  b=1  c=1  InitialConditionSource=internal  InitialConditionForIntegrator=0  InitialConditionForFilter=0  ExternalReset=none  LimitOutput=off  UpperSaturationLimit=inf  LowerSaturationLimit=-inf  LinearizeAsGain=off  AntiWindupMode=none  Kb=1  TrackingMode=off  Kt=1  PParamMin=[]  PParamMax=[]  IParamMin=[]  IParamMax=[]  DParamMin=[]  DParamMax=[]  NParamMin=[]  NParamMax=[]  bParamMin=[]  bParamMax=[]  cParamMin=[]  cParamMax=[]  KbParamMin=[]  KbParamMax=[]  KtParamMin=[]  KtParamMax=[]  POutMin=[]  POutMax=[]  IOutMin=[]  IOutMax=[]  DOutMin=[]  DOutMax=[]  NOutMin=[]  NOutMax=[]  bOutMin=[]  bOutMax=[]  cOutMin=[]  cOutMax=[]  KbOutMin=[]  KbOutMax=[]  KtOutMin=[]  KtOutMax=[]  IntegratorOutMin=[]  IntegratorOutMax=[]  FilterOutMin=[]  FilterOutMax=[]  SumOutMin=[]  SumOutMax=[]  Sum1OutMin=[]  Sum1OutMax=[]  Sum2OutMin=[]  Sum2OutMax=[]  Sum3OutMin=[]  Sum3OutMax=[]  SumI1OutMin=[]  SumI1OutMax=[]  SumI2OutMin=[]  SumI2OutMax=[]  SumI3OutMin=[]  SumI3OutMax=[]  SumDOutMin=[]  SumDOutMax=[]  SaturationOutMin=[]  SaturationOutMax=[]  IntegratorContinuousStateAttributes=''  IntegratorStateMustResolveToSignalObject=off  IntegratorRTWStateStorageClass=Auto  FilterContinuousStateAttributes=''  FilterStateMustResolveToSignalObject=off  FilterRTWStateStorageClass=Auto  DifferentiatorICPrevScaledInput=0  DifferentiatorOutMin=[]  DifferentiatorOutMax=[]  FilterDiffOutCoefMin=[]  FilterDiffOutCoefMax=[]  SumDenOutMin=[]  SumDenOutMax=[]  SumNumOutMin=[]  SumNumOutMax=[]  ReciprocalOutMin=[]  ReciprocalOutMax=[]  DivideOutMin=[]  DivideOutMax=[]  TunerSelectOption=Transfer Function Based (PID Tuner App)
  cfblk14 : Subsystem  TreatAsAtomicUnit=on
  cfblk3 : UnitDelay  SampleTime=-1
  cfblk4 : DiscreteTransferFcn
  cfblk5 : Subsystem  TreatAsAtomicUnit=on
  cfblk6 : Subsystem  TreatAsAtomicUnit=on
  cfblk7 : DiscreteFilter
  cfblk8 : Subsystem  TreatAsAtomicUnit=on
  cfblk9 : simulink/Discrete/Transfer Fcn Lead or Lag  PoleZ=0.95  ZeroZ=0.75  ICPrevOutput=0.0  ICPrevInput=0.0  DoSatur=off
      settings: SourceProductName=Simulink  SourceProductBaseCode=SL
  cyemi_{757..769} (13 alike) : DataTypeConversion  OutDataTypeStr=double
  emi_1059 : Subsystem  TreatAsAtomicUnit=on
  emi_{692,1061,1213,1376,1973} (5 alike) : If  IfExpression=Inf <= u1
  emi_{693,1062,1214,1377,1974} (5 alike) : DataTypeConversion  OutDataTypeStr=double
  emi_1211 : Subsystem  TreatAsAtomicUnit=on
  emi_1374 : Subsystem  TreatAsAtomicUnit=on
  emi_1971 : Subsystem  TreatAsAtomicUnit=on
  emi_690 : Subsystem  TreatAsAtomicUnit=on
  cfblk2 : Outport
  wires:
  cfblk1/1 -> cyemi_761/1, cyemi_767/1
  cyemi_758/1 -> cfblk11/1
  cyemi_759/1 -> cfblk12/1
  cfblk4/1 -> cyemi_759/1
  cyemi_760/1 -> cfblk13/1
  cfblk9/1 -> cyemi_760/1
  cyemi_761/1 -> cfblk13/2
  cfblk12/1 -> cyemi_762/1
  cyemi_763/1 -> cfblk3/1
  cfblk13/1 -> cyemi_763/1
  cyemi_764/1 -> cfblk4/1
  cfblk11/1 -> cyemi_764/1, emi_693/1, emi_1062/1, emi_1214/1, emi_1974/1
  cfblk7/1 -> cyemi_765/1
  cyemi_767/1 -> cfblk7/1
  cfblk3/1 -> cyemi_768/1, emi_1377/1
  cyemi_769/1 -> cfblk9/1
  cyemi_766/1 -> cfblk6/1(emi_688)
  cfblk6/1(emi_689) -> cyemi_769/1
  emi_692/1 -> cfblk6/Action
  emi_692/2 -> emi_690/Action
  emi_693/1 -> emi_692/1
  cyemi_757/1 -> cfblk10/1(emi_1057)
  cfblk10/1(emi_1058) -> cfblk2/1
  emi_1061/1 -> cfblk10/Action
  emi_1061/2 -> emi_1059/Action
  emi_1062/1 -> emi_1061/1
  cyemi_762/1 -> cfblk14/1(emi_1209)
  cfblk14/1(emi_1210) -> cyemi_766/1
  emi_1213/1 -> cfblk14/Action
  emi_1213/2 -> emi_1211/Action
  emi_1214/1 -> emi_1213/1
  cyemi_765/1 -> cfblk5/1(emi_1372)
  cfblk5/1(emi_1373) -> cyemi_758/1
  emi_1376/1 -> cfblk5/Action
  emi_1376/2 -> emi_1374/Action
  emi_1377/1 -> emi_1376/1
  cyemi_768/1 -> cfblk8/1(emi_1969)
  cfblk8/1(emi_1970) -> cyemi_757/1
  emi_1973/1 -> cfblk8/Action
  emi_1973/2 -> emi_1971/Action
  emi_1974/1 -> emi_1973/1

== system sampleModel7293_pp_1_1/cfblk190/emi_1802 ==
  Action Port : ActionPort  ActionType=else
  emi_1803 : Assertion

== system sampleModel7293_pp_1_1/cfblk190/emi_2028 ==
  Action Port : ActionPort  ActionType=else
  emi_2029 : Assertion

== system sampleModel7293_pp_1_1/cfblk190/emi_2142 ==
  Action Port : ActionPort  ActionType=else
  emi_2143 : Assertion

== system sampleModel7293_pp_1_1/cfblk190/emi_919 ==
  Action Port : ActionPort  ActionType=else
  emi_920 : Assertion

== system sampleModel7293_pp_1_1/cfblk191/cfblk5 ==
  emi_1216 : Inport
  Action Port : ActionPort  ActionType=then
  cfblk5 : simulink/Discrete/Transfer Fcn Real Zero  ZeroZ=0.75  ICPrevInput=0.0  DoSatur=off
      settings: SourceProductName=Simulink  SourceProductBaseCode=SL
  emi_1217 : Outport
  wires:
  emi_1216/1 -> cfblk5/1
  cfblk5/1 -> emi_1217/1

== system sampleModel7293_pp_1_1/cfblk191/emi_1218 ==
  Action Port : ActionPort  ActionType=else
  emi_1219 : Assertion

== system sampleModel7293_pp_1_1/cfblk193/cfblk10 ==
  emi_94 : Inport
  Action Port : ActionPort  ActionType=then
  cfblk10 : simulink/Discrete/Difference  ICPrevInput=0.0  OutMin=[]  OutMax=[]  OutDataTypeStr=double  OutputDataTypeScalingMode=double  OutDataType=fixdt(1, 16)  OutScaling=2^-10  DoSatur=off
  emi_95 : Outport
  wires:
  emi_94/1 -> cfblk10/1
  cfblk10/1 -> emi_95/1

== system sampleModel7293_pp_1_1/cfblk193/cfblk17 ==
  cfblk1 : Inport
  cfblk12 : Inport  Port=2
  cfblk13 : Inport  Port=3
  Action Port : ActionPort  ActionType=then
  cfblk10 : simulink/Discrete/Tapped Delay  vinit=0.0  samptime=-1  NumDelays=1  DelayOrder=Oldest  includeCurrent=off
  cfblk11 : DiscreteFilter
  cfblk3 : simulink/Discrete/Transfer Fcn Lead or Lag  PoleZ=0.95  ZeroZ=0.75  ICPrevOutput=0.0  ICPrevInput=0.0  DoSatur=off
      settings: SourceProductName=Simulink  SourceProductBaseCode=SL
  cfblk4 : Delay
  cfblk5 : DiscreteTransferFcn
  cfblk6 : Subsystem  TreatAsAtomicUnit=on
  cfblk7 : simulink/Discrete/Difference  ICPrevInput=0.0  OutMin=[]  OutMax=[]  OutDataTypeStr=double  OutputDataTypeScalingMode=double  OutDataType=fixdt(1, 16)  OutScaling=2^-10  DoSatur=off
  cfblk8 : Subsystem  TreatAsAtomicUnit=on
  cfblk9 : UnitDelay  SampleTime=-1
  cyemi_{801..809} (9 alike) : DataTypeConversion  OutDataTypeStr=double
  emi_2056 : Subsystem  TreatAsAtomicUnit=on
  emi_2058 : If  IfExpression=Inf <= u1
  emi_2059 : DataTypeConversion  OutDataTypeStr=double
  emi_24 : Subsystem  TreatAsAtomicUnit=on
  emi_26 : If  IfExpression=Inf <= u1
  emi_27 : DataTypeConversion  OutDataTypeStr=double
  cfblk2 : Outport
  cfblk14 : Outport  Port=2
  wires:
  cyemi_801/1 -> cfblk10/1
  cfblk1/1 -> cyemi_801/1
  cyemi_802/1 -> cfblk11/1
  cfblk5/1 -> cyemi_802/1, emi_27/1
  cyemi_803/1 -> cfblk3/1
  cfblk7/1 -> cyemi_803/1
  cyemi_804/1 -> cfblk4/1
  cfblk3/1 -> cyemi_804/1
  cyemi_805/1 -> cfblk5/1
  cfblk12/1 -> cyemi_805/1
  cfblk9/1 -> cyemi_806/1
  cyemi_807/1 -> cfblk7/1
  cfblk11/1 -> cyemi_807/1, emi_2059/1
  cfblk10/1 -> cyemi_808/1
  cyemi_809/1 -> cfblk9/1
  cfblk13/1 -> cyemi_809/1
  cyemi_808/1 -> cfblk8/1(emi_22)
  cfblk8/1(emi_23) -> cfblk2/1
  emi_26/1 -> cfblk8/Action
  emi_26/2 -> emi_24/Action
  emi_27/1 -> emi_26/1
  cyemi_806/1 -> cfblk6/1(emi_2054)
  cfblk6/1(emi_2055) -> cfblk14/1
  emi_2058/1 -> cfblk6/Action
  emi_2058/2 -> emi_2056/Action
  emi_2059/1 -> emi_2058/1

== system sampleModel7293_pp_1_1/cfblk193/cfblk18 ==
  cfblk1 : Inport
  cfblk11 : Inport  Port=2
  Action Port : ActionPort  ActionType=else
  cfblk10 : simulink/Continuous/PID Controller  Controller=PID  TimeDomain=Discrete-time  SampleTime=-1  IntegratorMethod=Forward Euler  FilterMethod=Forward Euler  Form=Parallel  UseFilter=on  ControllerParametersSource=internal  P=1  I=1  D=0  N=100  InitialConditionSource=internal  InitialConditionForIntegrator=0  InitialConditionForFilter=0  ExternalReset=none  LimitOutput=off  UpperSaturationLimit=inf  LowerSaturationLimit=-inf  LinearizeAsGain=off  AntiWindupMode=none  Kb=1  TrackingMode=off  Kt=1  PParamMin=[]  PParamMax=[]  IParamMin=[]  IParamMax=[]  DParamMin=[]  DParamMax=[]  NParamMin=[]  NParamMax=[]  KbParamMin=[]  KbParamMax=[]  KtParamMin=[]  KtParamMax=[]  POutMin=[]  POutMax=[]  IOutMin=[]  IOutMax=[]  DOutMin=[]  DOutMax=[]  NOutMin=[]  NOutMax=[]  KbOutMin=[]  KbOutMax=[]  KtOutMin=[]  KtOutMax=[]  IntegratorOutMin=[]  IntegratorOutMax=[]  FilterOutMin=[]  FilterOutMax=[]  SumOutMin=[]  SumOutMax=[]  SumI1OutMin=[]  SumI1OutMax=[]  SumI2OutMin=[]  SumI2OutMax=[]  SumI3OutMin=[]  SumI3OutMax=[]  SumDOutMin=[]  SumDOutMax=[]  SaturationOutMin=[]  SaturationOutMax=[]  IntegratorContinuousStateAttributes=''  IntegratorStateMustResolveToSignalObject=off  IntegratorRTWStateStorageClass=Auto  FilterContinuousStateAttributes=''  FilterStateMustResolveToSignalObject=off  FilterRTWStateStorageClass=Auto  DifferentiatorICPrevScaledInput=0  DifferentiatorOutMin=[]  DifferentiatorOutMax=[]  FilterDiffOutCoefMin=[]  FilterDiffOutCoefMax=[]  SumDenOutMin=[]  SumDenOutMax=[]  SumNumOutMin=[]  SumNumOutMax=[]  ReciprocalOutMin=[]  ReciprocalOutMax=[]  DivideOutMin=[]  DivideOutMax=[]  TunerSelectOption=Transfer Function Based (PID Tuner App)
  cfblk12 : Delay
  cfblk3 : simulink/Discrete/Transfer Fcn First Order  PoleZ=0.95  ICPrevOutput=0.0  DoSatur=off
      settings: SourceProductName=Simulink
  cfblk4 : simulink/Discrete/Transfer Fcn Lead or Lag  PoleZ=0.95  ZeroZ=0.75  ICPrevOutput=0.0  ICPrevInput=0.0  DoSatur=off
      settings: SourceProductName=Simulink  SourceProductBaseCode=SL
  cfblk5 : DiscreteIntegrator  SampleTime=-1  OutDataTypeStr=double  ICPrevOutput=DiscIntNeverNeededParam  ICPrevScaledInput=DiscIntNeverNeededParam
  cfblk6 : Delay  ShowEnablePort=on
      settings: InputPortMap=u0,e6
  cfblk7 : UnitDelay  SampleTime=-1
  cfblk8 : simulink/Discrete/Tapped Delay  vinit=0.0  samptime=-1  NumDelays=1  DelayOrder=Oldest  includeCurrent=off
  cfblk9 : simulink/Continuous/PID Controller (2DOF)  Controller=PID  TimeDomain=Discrete-time  SampleTime=-1  IntegratorMethod=Forward Euler  FilterMethod=Forward Euler  Form=Parallel  UseFilter=on  ControllerParametersSource=internal  P=1  I=1  D=0  N=100  b=1  c=1  InitialConditionSource=internal  InitialConditionForIntegrator=0  InitialConditionForFilter=0  ExternalReset=none  LimitOutput=off  UpperSaturationLimit=inf  LowerSaturationLimit=-inf  LinearizeAsGain=off  AntiWindupMode=none  Kb=1  TrackingMode=off  Kt=1  PParamMin=[]  PParamMax=[]  IParamMin=[]  IParamMax=[]  DParamMin=[]  DParamMax=[]  NParamMin=[]  NParamMax=[]  bParamMin=[]  bParamMax=[]  cParamMin=[]  cParamMax=[]  KbParamMin=[]  KbParamMax=[]  KtParamMin=[]  KtParamMax=[]  POutMin=[]  POutMax=[]  IOutMin=[]  IOutMax=[]  DOutMin=[]  DOutMax=[]  NOutMin=[]  NOutMax=[]  bOutMin=[]  bOutMax=[]  cOutMin=[]  cOutMax=[]  KbOutMin=[]  KbOutMax=[]  KtOutMin=[]  KtOutMax=[]  IntegratorOutMin=[]  IntegratorOutMax=[]  FilterOutMin=[]  FilterOutMax=[]  SumOutMin=[]  SumOutMax=[]  Sum1OutMin=[]  Sum1OutMax=[]  Sum2OutMin=[]  Sum2OutMax=[]  Sum3OutMin=[]  Sum3OutMax=[]  SumI1OutMin=[]  SumI1OutMax=[]  SumI2OutMin=[]  SumI2OutMax=[]  SumI3OutMin=[]  SumI3OutMax=[]  SumDOutMin=[]  SumDOutMax=[]  SaturationOutMin=[]  SaturationOutMax=[]  IntegratorContinuousStateAttributes=''  IntegratorStateMustResolveToSignalObject=off  IntegratorRTWStateStorageClass=Auto  FilterContinuousStateAttributes=''  FilterStateMustResolveToSignalObject=off  FilterRTWStateStorageClass=Auto  DifferentiatorICPrevScaledInput=0  DifferentiatorOutMin=[]  DifferentiatorOutMax=[]  FilterDiffOutCoefMin=[]  FilterDiffOutCoefMax=[]  SumDenOutMin=[]  SumDenOutMax=[]  SumNumOutMin=[]  SumNumOutMax=[]  ReciprocalOutMin=[]  ReciprocalOutMax=[]  DivideOutMin=[]  DivideOutMax=[]  TunerSelectOption=Transfer Function Based (PID Tuner App)
  cyemi_{812..822} (11 alike) : DataTypeConversion  OutDataTypeStr=double
  cfblk2 : Outport
  wires:
  cfblk8/1 -> cfblk2/1
  cfblk1/1 -> cyemi_816/1, cyemi_817/1
  cfblk11/1 -> cyemi_818/1, cyemi_822/1
  cyemi_812/1 -> cfblk10/1
  cfblk4/1 -> cyemi_812/1
  cyemi_813/1 -> cfblk12/1
  cfblk9/1 -> cyemi_813/1
  cyemi_814/1 -> cfblk3/1
  cfblk10/1 -> cyemi_814/1
  cyemi_815/1 -> cfblk4/1
  cfblk5/1 -> cyemi_815/1
  cyemi_816/1 -> cfblk5/1
  cyemi_817/1 -> cfblk6/1
  cyemi_818/1 -> cfblk6/2
  cyemi_819/1 -> cfblk7/1
  cfblk12/1 -> cyemi_819/1
  cyemi_820/1 -> cfblk8/1
  cfblk3/1 -> cyemi_820/1
  cyemi_821/1 -> cfblk9/1
  cfblk7/1 -> cyemi_821/1
  cyemi_822/1 -> cfblk9/2

== system sampleModel7293_pp_1_1/cfblk193/cfblk19 ==
  cfblk1 : Inport
  cfblk13 : Inport  Port=2
  cfblk14 : Inport  Port=3
  Action Port : ActionPort  ActionType=then
  cfblk10 : DiscreteFilter
  cfblk11 : simulink/Discrete/Tapped Delay  vinit=0.0  samptime=-1  NumDelays=1  DelayOrder=Oldest  includeCurrent=off
  cfblk12 : simulink/Discrete/Transfer Fcn Real Zero  ZeroZ=0.75  ICPrevInput=0.0  DoSatur=off
      settings: SourceProductName=Simulink  SourceProductBaseCode=SL
  cfblk17 : Delay
  cfblk18 : Subsystem  TreatAsAtomicUnit=on
  cfblk19 : Delay
  cfblk3 : simulink/Continuous/PID Controller (2DOF)  Controller=PID  TimeDomain=Discrete-time  SampleTime=-1  IntegratorMethod=Forward Euler  FilterMethod=Forward Euler  Form=Parallel  UseFilter=on  ControllerParametersSource=internal  P=1  I=1  D=0  N=100  b=1  c=1  InitialConditionSource=internal  InitialConditionForIntegrator=0  InitialConditionForFilter=0  ExternalReset=none  LimitOutput=off  UpperSaturationLimit=inf  LowerSaturationLimit=-inf  LinearizeAsGain=off  AntiWindupMode=none  Kb=1  TrackingMode=off  Kt=1  PParamMin=[]  PParamMax=[]  IParamMin=[]  IParamMax=[]  DParamMin=[]  DParamMax=[]  NParamMin=[]  NParamMax=[]  bParamMin=[]  bParamMax=[]  cParamMin=[]  cParamMax=[]  KbParamMin=[]  KbParamMax=[]  KtParamMin=[]  KtParamMax=[]  POutMin=[]  POutMax=[]  IOutMin=[]  IOutMax=[]  DOutMin=[]  DOutMax=[]  NOutMin=[]  NOutMax=[]  bOutMin=[]  bOutMax=[]  cOutMin=[]  cOutMax=[]  KbOutMin=[]  KbOutMax=[]  KtOutMin=[]  KtOutMax=[]  IntegratorOutMin=[]  IntegratorOutMax=[]  FilterOutMin=[]  FilterOutMax=[]  SumOutMin=[]  SumOutMax=[]  Sum1OutMin=[]  Sum1OutMax=[]  Sum2OutMin=[]  Sum2OutMax=[]  Sum3OutMin=[]  Sum3OutMax=[]  SumI1OutMin=[]  SumI1OutMax=[]  SumI2OutMin=[]  SumI2OutMax=[]  SumI3OutMin=[]  SumI3OutMax=[]  SumDOutMin=[]  SumDOutMax=[]  SaturationOutMin=[]  SaturationOutMax=[]  IntegratorContinuousStateAttributes=''  IntegratorStateMustResolveToSignalObject=off  IntegratorRTWStateStorageClass=Auto  FilterContinuousStateAttributes=''  FilterStateMustResolveToSignalObject=off  FilterRTWStateStorageClass=Auto  DifferentiatorICPrevScaledInput=0  DifferentiatorOutMin=[]  DifferentiatorOutMax=[]  FilterDiffOutCoefMin=[]  FilterDiffOutCoefMax=[]  SumDenOutMin=[]  SumDenOutMax=[]  SumNumOutMin=[]  SumNumOutMax=[]  ReciprocalOutMin=[]  ReciprocalOutMax=[]  DivideOutMin=[]  DivideOutMax=[]  TunerSelectOption=Transfer Function Based (PID Tuner App)
  cfblk4 : Delay  ShowEnablePort=on
      settings: InputPortMap=u0,e6
  cfblk5 : simulink/Discrete/Tapped Delay  vinit=0.0  samptime=-1  NumDelays=1  DelayOrder=Oldest  includeCurrent=off
  cfblk6 : simulink/Discrete/Transfer Fcn Real Zero  ZeroZ=0.75  ICPrevInput=0.0  DoSatur=off
      settings: SourceProductName=Simulink  SourceProductBaseCode=SL
  cfblk7 : simulink/Discrete/Transfer Fcn Lead or Lag  PoleZ=0.95  ZeroZ=0.75  ICPrevOutput=0.0  ICPrevInput=0.0  DoSatur=off
      settings: SourceProductName=Simulink  SourceProductBaseCode=SL
  cfblk8 : simulink/Continuous/PID Controller (2DOF)  Controller=PID  TimeDomain=Discrete-time  SampleTime=-1  IntegratorMethod=Forward Euler  FilterMethod=Forward Euler  Form=Parallel  UseFilter=on  ControllerParametersSource=internal  P=1  I=1  D=0  N=100  b=1  c=1  InitialConditionSource=internal  InitialConditionForIntegrator=0  InitialConditionForFilter=0  ExternalReset=none  LimitOutput=off  UpperSaturationLimit=inf  LowerSaturationLimit=-inf  LinearizeAsGain=off  AntiWindupMode=none  Kb=1  TrackingMode=off  Kt=1  PParamMin=[]  PParamMax=[]  IParamMin=[]  IParamMax=[]  DParamMin=[]  DParamMax=[]  NParamMin=[]  NParamMax=[]  bParamMin=[]  bParamMax=[]  cParamMin=[]  cParamMax=[]  KbParamMin=[]  KbParamMax=[]  KtParamMin=[]  KtParamMax=[]  POutMin=[]  POutMax=[]  IOutMin=[]  IOutMax=[]  DOutMin=[]  DOutMax=[]  NOutMin=[]  NOutMax=[]  bOutMin=[]  bOutMax=[]  cOutMin=[]  cOutMax=[]  KbOutMin=[]  KbOutMax=[]  KtOutMin=[]  KtOutMax=[]  IntegratorOutMin=[]  IntegratorOutMax=[]  FilterOutMin=[]  FilterOutMax=[]  SumOutMin=[]  SumOutMax=[]  Sum1OutMin=[]  Sum1OutMax=[]  Sum2OutMin=[]  Sum2OutMax=[]  Sum3OutMin=[]  Sum3OutMax=[]  SumI1OutMin=[]  SumI1OutMax=[]  SumI2OutMin=[]  SumI2OutMax=[]  SumI3OutMin=[]  SumI3OutMax=[]  SumDOutMin=[]  SumDOutMax=[]  SaturationOutMin=[]  SaturationOutMax=[]  IntegratorContinuousStateAttributes=''  IntegratorStateMustResolveToSignalObject=off  IntegratorRTWStateStorageClass=Auto  FilterContinuousStateAttributes=''  FilterStateMustResolveToSignalObject=off  FilterRTWStateStorageClass=Auto  DifferentiatorICPrevScaledInput=0  DifferentiatorOutMin=[]  DifferentiatorOutMax=[]  FilterDiffOutCoefMin=[]  FilterDiffOutCoefMax=[]  SumDenOutMin=[]  SumDenOutMax=[]  SumNumOutMin=[]  SumNumOutMax=[]  ReciprocalOutMin=[]  ReciprocalOutMax=[]  DivideOutMin=[]  DivideOutMax=[]  TunerSelectOption=Transfer Function Based (PID Tuner App)
  cfblk9 : UnitDelay  SampleTime=-1
  cyemi_{826..841} (16 alike) : DataTypeConversion  OutDataTypeStr=double
  emi_697 : Subsystem  TreatAsAtomicUnit=on
  emi_699 : If  IfExpression=0 <= u1
  emi_700 : DataTypeConversion  OutDataTypeStr=double
  cfblk2 : Outport
  cfblk15 : Outport  Port=2
  cfblk16 : Outport  Port=3
  wires:
  cfblk10/1 -> cfblk2/1, cyemi_828/1
  cfblk11/1 -> cyemi_830/1, cyemi_841/1
  cfblk1/1 -> cfblk16/1
  cfblk8/1 -> cfblk15/1, cyemi_826/1
  cyemi_826/1 -> cfblk10/1
  cyemi_827/1 -> cfblk11/1
  cfblk12/1 -> cyemi_827/1
  cyemi_828/1 -> cfblk12/1
  cyemi_829/1 -> cfblk17/1
  cfblk5/1 -> cyemi_829/1
  cyemi_831/1 -> cfblk19/1
  cfblk9/1 -> cyemi_831/1
  cyemi_832/1 -> cfblk3/1
  cfblk17/1 -> cyemi_832/1
  cyemi_833/1 -> cfblk3/2
  cfblk13/1 -> cyemi_833/1
  cyemi_834/1 -> cfblk4/1
  cfblk7/1 -> cyemi_834/1
  cyemi_835/1 -> cfblk4/2
  cfblk19/1 -> cyemi_835/1, emi_700/1
  cyemi_836/1 -> cfblk5/1
  cfblk3/1 -> cyemi_836/1
  cyemi_837/1 -> cfblk6/1
  cfblk14/1 -> cyemi_837/1
  cyemi_838/1 -> cfblk7/1
  cfblk6/1 -> cyemi_838/1
  cyemi_839/1 -> cfblk8/1
  cyemi_840/1 -> cfblk8/2
  cfblk4/1 -> cyemi_840/1
  cyemi_841/1 -> cfblk9/1
  cyemi_830/1 -> cfblk18/1(emi_695)
  cfblk18/1(emi_696) -> cyemi_839/1
  emi_699/1 -> cfblk18/Action
  emi_699/2 -> emi_697/Action
  emi_700/1 -> emi_699/1

== system sampleModel7293_pp_1_1/cfblk193/cfblk20 ==
  cfblk1 : Inport
  cfblk13 : Inport  Port=2
  cfblk14 : Inport  Port=3
  Action Port : ActionPort  ActionType=else
  cfblk10 : Subsystem  TreatAsAtomicUnit=on
  cfblk11 : DiscreteStateSpace  SampleTime=-1
  cfblk12 : DiscreteFilter
  cfblk3 : DiscreteFilter
  cfblk4 : Subsystem  TreatAsAtomicUnit=on
  cfblk5 : DiscreteZeroPole  Poles=[0 0.5]  Gain=1  SampleTime=-1
  cfblk6 : Delay  ShowEnablePort=on
      settings: InputPortMap=u0,e6
  cfblk7 : Subsystem  TreatAsAtomicUnit=on
  cfblk8 : simulink/Discrete/Tapped Delay  vinit=0.0  samptime=-1  NumDelays=1  DelayOrder=Oldest  includeCurrent=off
  cfblk9 : DiscreteIntegrator  SampleTime=-1  OutDataTypeStr=double  ICPrevOutput=DiscIntNeverNeededParam  ICPrevScaledInput=DiscIntNeverNeededParam
  cyemi_{845..855} (11 alike) : DataTypeConversion  OutDataTypeStr=double
  emi_224 : Subsystem  TreatAsAtomicUnit=on
  emi_226 : If  IfExpression=0 <= u1
  emi_227 : DataTypeConversion  OutDataTypeStr=double
  emi_540 : Subsystem  TreatAsAtomicUnit=on
  emi_542 : If  IfExpression=0 <= u1
  emi_543 : DataTypeConversion  OutDataTypeStr=double
  emi_612 : Subsystem  TreatAsAtomicUnit=on
  emi_614 : If  IfExpression=0 <= u1
  emi_615 : DataTypeConversion  OutDataTypeStr=double
  cfblk2 : Outport
  cfblk15 : Outport  Port=2
  cfblk16 : Outport  Port=3
  wires:
  cfblk6/1 -> cfblk2/1, emi_543/1
  cfblk13/1 -> cfblk15/1
  cfblk9/1 -> cfblk16/1, cyemi_850/1
  cfblk12/1 -> cyemi_845/1
  cyemi_846/1 -> cfblk11/1
  cyemi_847/1 -> cfblk12/1
  cfblk8/1 -> cyemi_847/1
  cyemi_848/1 -> cfblk3/1
  cfblk5/1 -> cyemi_849/1
  cyemi_850/1 -> cfblk5/1
  cyemi_851/1 -> cfblk6/1
  cfblk11/1 -> cyemi_851/1
  cyemi_852/1 -> cfblk6/2
  cfblk1/1 -> cyemi_853/1
  cyemi_854/1 -> cfblk8/1
  cfblk14/1 -> cyemi_854/1
  cyemi_855/1 -> cfblk9/1
  cfblk3/1 -> cyemi_855/1
  cyemi_849/1 -> cfblk4/1(emi_222)
  cfblk4/1(emi_223) -> cyemi_852/1
  emi_226/1 -> cfblk4/Action
  emi_226/2 -> emi_224/Action
  emi_227/1 -> emi_226/1
  cyemi_845/1 -> cfblk10/1(emi_538)
  cfblk10/1(emi_539) -> cyemi_848/1, emi_615/1
  emi_542/1 -> cfblk10/Action
  emi_542/2 -> emi_540/Action
  emi_543/1 -> emi_542/1
  cyemi_853/1 -> cfblk7/1(emi_610)
  cfblk7/1(emi_611) -> emi_227/1, cyemi_846/1
  emi_614/1 -> cfblk7/Action
  emi_614/2 -> emi_612/Action
  emi_615/1 -> emi_614/1

== system sampleModel7293_pp_1_1/cfblk193/cfblk24 ==
  emi_201 : Inport
  Action Port : ActionPort  ActionType=then
  cfblk24 : Delay
  emi_202 : Outport
  wires:
  emi_201/1 -> cfblk24/1
  cfblk24/1 -> emi_202/1

== system sampleModel7293_pp_1_1/cfblk193/emi_203 ==
  Action Port : ActionPort  ActionType=else
  emi_204 : Assertion

== system sampleModel7293_pp_1_1/cfblk193/emi_96 ==
  Action Port : ActionPort  ActionType=else
  emi_97 : Assertion
